simulink model "ac3"  (R2013a)
settings: Solver=VariableStepDiscrete  StartTime=0.0  StopTime=stime  RelTol=1e-3
values from neighbouring files (symbols this model uses):
  Fsour = 60    [matlab.mat]    (also in sim5.m)
  poles = 2    [matlab.mat]    (also in sim5.m)
  stime = 9    [matlab.mat]    (also in sim5.m)
  t1 = 1    [sim5.m]
  t2 = 4    [sim5.m]
  ti = 1    [matlab.mat]    (also in sim5.m = 0)
  tt = 6    [matlab.mat]    (also in sim5.m)
  Vsour = 220    [matlab.mat]    (also in sim5.m)
  wref = 1500    [matlab.mat]    (also in sim5.m)
libraries: powerlib x2, powerlib_meascontrol x1, simulink x1, electricdrivelib x1
settings Model: Creator=dello  LastModifiedBy=dello
settings SolverCC: SolverResetMethod=Robust
settings DataIOCC: SignalLoggingSaveFormat=ModelDataLogs  SignalLoggingName=results
settings OptimizationCC: BlockReduction=off
settings DebuggingCC: UnconnectedInputMsg=none  UnconnectedOutputMsg=none  UnconnectedLineMsg=none

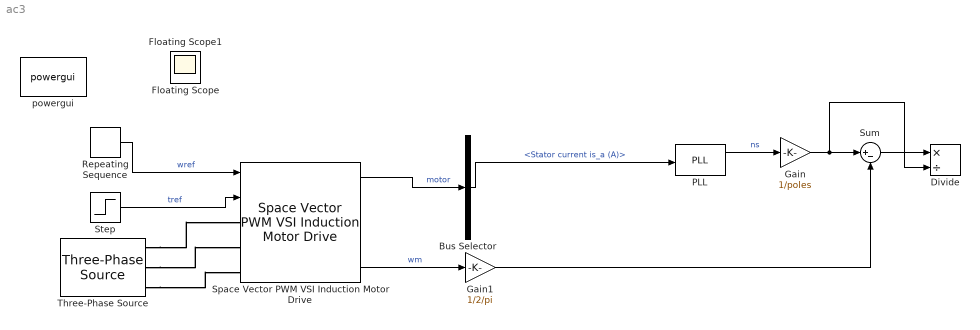
== system ac3 ==
  Bus Selector : BusSelector  OutputSignals=Stator measurements.Stator current is_a (A)
  Divide : Product  Inputs=*/
  Gain : Gain  Gain=1/poles
  Gain1 : Gain  Gain=1/2/pi
  PLL : powerlib_meascontrol/PLL/PLL  Fmin=25  Par_Init=[0, 25]  ParK=[180, 3200, 1]  TcD=1e-4  MaxRateChangeFreq=120  FilterCutOffFreq=15  Ts=1e-5  AGC=on
  Repeating Sequence : simulink/Sources/Repeating Sequence  rep_seq_t=[0 t1 t2 stime]  rep_seq_y="[0 0 wref  wref]"
  Space Vector PWM VSI Induction Motor Drive : electricdrivelib/AC drives/Space Vector PWM VSI Induction Motor Drive  showMaskWarnings=on  AverageValue=off  MechanicalLoad=Torque Tm  driveType=AC2
  Step : Step  Time=tt  Before=ti  After=tf  SampleTime=0
  Sum : Sum  Inputs=|+-
  Three-Phase Source : powerlib/Electrical Sources/Three-Phase Source  Voltage=Vsour  PhaseAngle=0  Frequency=Fsour  InternalConnection=Yg  SpecifyImpedance=on  Resistance=0.8929  Inductance=16.58e-3  ShortCircuitLevel=100e6  BaseVoltage=25e3  XRratio=7  BusType=swing  Pref=0  Qref=0  Qmin=-inf  Qmax=inf
  powergui : powerlib/powergui  Priority=1  SimulationMode=Discrete  SolverType=Backward Euler  SampleTime=1e-5  frequency=60  SPID=off  DisableSnubberDevices=off  DisableRonSwitches=off  DisableVfSwitches=off  SwTol=0  Interpol=off  DisplayEquations=off  frequencyindice=60  Pbase=100e6  ErrMax=1e-4  Iterations=50  UnitsV=kV  UnitsW=MW  FunctionMessages=off  echomessages=off  HookPort=off  EnableUseOfTLC=off  x0status=blocks  RestoreLinks=warning  ResistiveCurrentMeasurement=off  Frange=[0:2:500]  Ylog=off  Xlog=on  ShowGrid=off  save=off  variable=ZData  ZoomFFT=off  StartTime=0.0  cycles=1  DisplayStyle=1  fundamental=60  FreqAxis=off  MaxFrequency=1000  frequencyindicesteady=1  RmsSteady=1  display=off  Ts=0  methode=off
  Floating Scope : Scope  NumInputPorts=8
      settings: Floating=on  TimeRange=0.03333333333333333  YMin=-5~-5~-5~-5~-5~-5~-5~-5  YMax=5~5~5~5~5~5~5~5  SaveName=diodes
  Floating Scope1 : Scope
      settings: Floating=on  TimeRange=0.03333333333333333  SaveName=simdata
  wires:
  Step/1 -> Space Vector PWM VSI Induction Motor Drive/2  "tref"
  Repeating Sequence/1 -> Space Vector PWM VSI Induction Motor Drive/1  "wref"
  Space Vector PWM VSI Induction Motor Drive/1 -> Bus Selector/1  "motor"
  Bus Selector/1 -> PLL/1  "<Stator current is_a (A)>"
  PLL/1 -> Gain/1  "ns"
  Gain/1 -> Divide/2, Sum/1
  Space Vector PWM VSI Induction Motor Drive/4 -> Gain1/1  "wm"
  Gain1/1 -> Sum/2
  Sum/1 -> Divide/1
  connections:
  Three-Phase Source/RConn1 -- Space Vector PWM VSI Induction Motor Drive/LConn1
  Three-Phase Source/RConn2 -- Space Vector PWM VSI Induction Motor Drive/LConn2
  Three-Phase Source/RConn3 -- Space Vector PWM VSI Induction Motor Drive/LConn3
